simulink subsystem "PieroControladoV"  (R2023b)
settings: Solver=VariableStepAuto  StartTime=0.0  StopTime=10.0  RelTol=1e-3
settings Model: Creator=ricfe  LastModifiedBy=ricfe

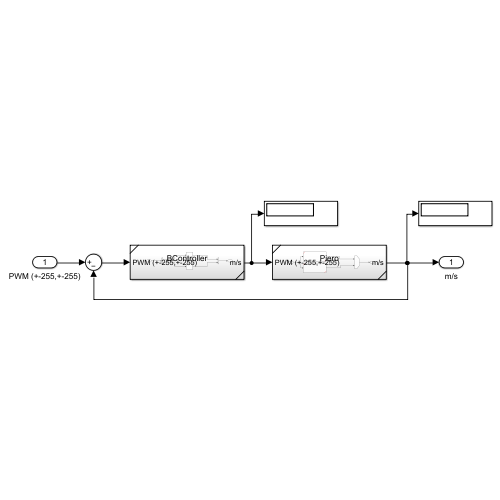
[thumbnail: Simulink's stored preview of the top-level diagram]
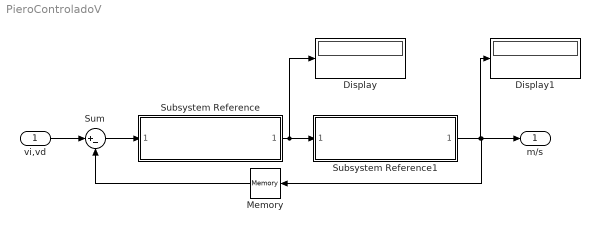
== system PieroControladoV ==
  vi,vd : Inport
  Display : Display
  Display1 : Display
  Memory : Memory
  Subsystem Reference : Subsystem  ReferencedSubsystem=BController
  Subsystem Reference1 : Subsystem  ReferencedSubsystem=Piero
  Sum : Sum  Inputs=|+-
  m/s : Outport
  wires:
  Subsystem Reference/1 -> Display/1, Subsystem Reference1/1
  Subsystem Reference1/1 -> Display1/1, m/s/1, Memory/1
  Sum/1 -> Subsystem Reference/1
  vi,vd/1 -> Sum/1
  Memory/1 -> Sum/2
